simulink model "time_to_frequency_domain_cosines_1"  (R2020b)
settings: Solver=FixedStepDiscrete  StartTime=0.0  StopTime=2  RelTol=1e-3
PreLoadFcn:
  | fs=2^14
InitFcn:
  | %fs=350*3
  | fs=2^14
undefined symbols (not defined in the file or in its folder): startfcn_spectrum_analyzer
settings Model: Creator=cmuller  LastModifiedBy=cmuller
settings SolverCC: AutoInsertRateTranBlk=on
settings DataIOCC: LimitDataPoints=on  SaveOutput=off  SignalLogging=off  SaveTime=off
settings OptimizationCC: LifeSpan=inf  SimCompilerOptimization=on
settings DebuggingCC: AlgebraicLoopMsg=error  SingleTaskRateTransMsg=error  AllowSymbolicDim=off  SFUnexpectedBacktrackingDiag=warning  SFNoUnconditionalDefaultTransitionDiag=warning  SFExecutionAtInitializationDiag=none  ArithmeticOperatorsInVariantConditions=warning
settings SFSimCC: SimUseLocalCustomCode=off  CustomCodeUndefinedFunction=UseInterfaceOnly
settings RTWCC: RTWUseLocalCustomCode=off
settings CodeAppCC: StateflowObjectComments=on
settings GRTTargetCC: TargetLangStandard=C89/C90 (ANSI)
settings ConfigComp: CovMetricSettings=dw  CovSaveCumulativeToWorkspaceVar=on  CovSaveSingleToWorkspaceVar=on  CovExternalEMLEnable=off  CovSFcnEnable=off

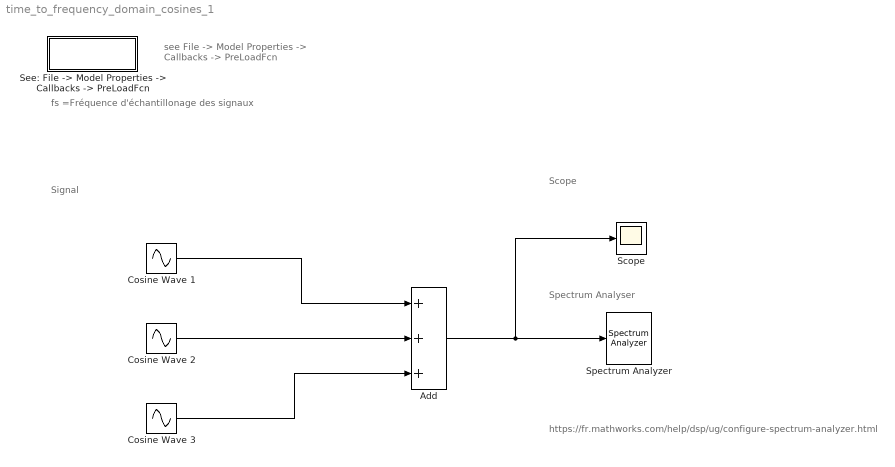
== system time_to_frequency_domain_cosines_1 ==
  note: https://fr.mathworks.com/help/dsp/ug/configure-spectrum-analyzer.html
  note: fs =Fréquence d'échantillonage des signaux
  note: Signal
  note: Scope
  note: see File -> Model Properties
      | -> Callbacks -> PreLoadFcn
  note: Spectrum Analyser
  Add : Sum  Inputs=+++
  Cosine Wave 1 : Sin  Amplitude=10  Frequency=2*pi*128  Phase=pi/2  SampleTime=1/fs
  Cosine Wave 2 : Sin  Frequency=2*pi*320  Phase=pi/2  SampleTime=1/fs
  Cosine Wave 3 : Sin  Amplitude=4  Frequency=2*pi*512  Phase=pi/2  SampleTime=1/fs
  "Scope " : Scope
      settings: Tag=Scope
  "See: File -> Model Properties -> Callbacks -> PreLoadFcn " : Subsystem
      mask Display:
      | fs = evalin('base', 'fs');
      | fprintf(['fs = ',num2str(fs),' Hz']);
  Spectrum Analyzer : SpectrumAnalyzer  Tag=Spectrum Analyser  StartFcn=startfcn_spectrum_analyzer;
  wires:
  Cosine Wave 1/1 -> Add/1
  Cosine Wave 3/1 -> Add/3
  Add/1 -> "Scope "/1, Spectrum Analyzer/1
  Cosine Wave 2/1 -> Add/2

== system time_to_frequency_domain_cosines_1/See: File -> Model Properties -> Callbacks -> PreLoadFcn  ==
